simulink model "Two_Wheel_PI"  (R2021b)
settings: Solver=VariableStepAuto  StartTime=0.0  StopTime=10.0  RelTol=1e-3
model workspace (MAT data in the model file):
  Ki = 3
  Kp = 1
  ic = [0 0 0 0 0 0]
  param = [9.81 0.05 0.2 0.2 0.1 0.01 0.01 1 1 1 1 1 1]
undefined symbols (not defined in the file or in its folder): B_s
settings Model: Creator=Lorenzo  LastModifiedBy=Lorenzo

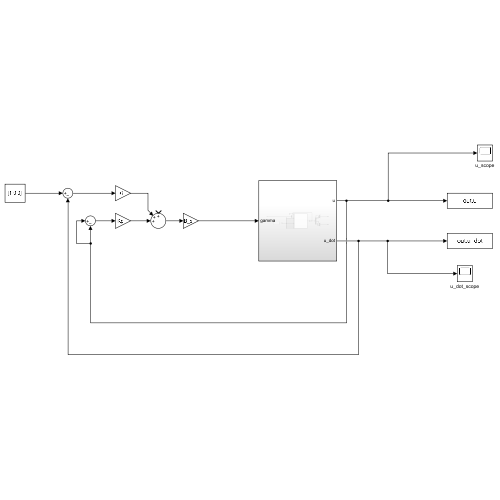
[thumbnail: Simulink's stored preview of the top-level diagram]
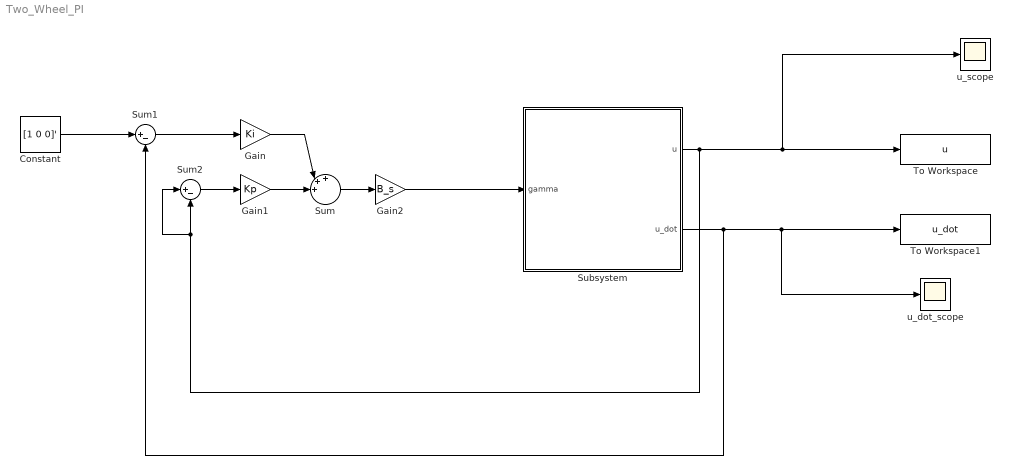
== system Two_Wheel_PI ==
  Constant : Constant  Value=[1 0 0]'
  Gain : Gain  Gain=Ki
  Gain1 : Gain  Gain=Kp
  Gain2 : Gain  Gain=B_s
  Subsystem : Subsystem
  Sum : Sum  Inputs=+++||
  Sum1 : Sum  Inputs=|+-
  Sum2 : Sum  Inputs=|+-
  To Workspace : ToWorkspace  VariableName=u  SaveFormat=Timeseries  SampleTime=-1
  To Workspace1 : ToWorkspace  VariableName=u_dot  SaveFormat=Timeseries  SampleTime=-1
  u_dot_scope : Scope
  u_scope : Scope
  wires:
  Subsystem/2(u_dot) -> u_dot_scope/1, To Workspace1/1, Sum1/2
  Subsystem/1(u) -> To Workspace/1, u_scope/1, Sum2/1, Sum2/2
  Gain2/1 -> Subsystem/1(gamma)
  Sum/1 -> Gain2/1
  Gain1/1 -> Sum/3
  Gain/1 -> Sum/2
  Sum1/1 -> Gain/1
  Sum2/1 -> Gain1/1
  Constant/1 -> Sum1/1

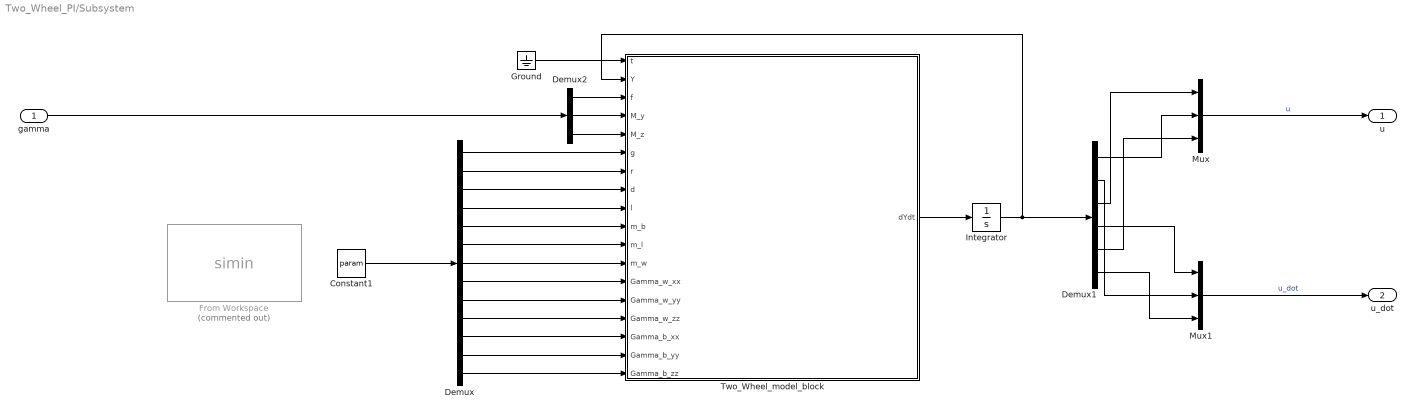
== system Two_Wheel_PI/Subsystem ==
  gamma : Inport
  Constant1 : Constant  Value=param
  Demux : Demux  Outputs=13
  Demux1 : Demux  Outputs=6
  Demux2 : Demux  Outputs=3
  From Workspace : FromWorkspace  Commented=on  VariableName=simin
  Ground : Ground
  Integrator : Integrator  InitialCondition=ic
  Mux : Mux  Inputs=3
  Mux1 : Mux  Inputs=3
  Two_Wheel_model_block : MATLAB Function  TreatAsAtomicUnit=on
  u : Outport
  u_dot : Outport  Port=2
  wires:
  Demux/9 -> Two_Wheel_model_block/14(Gamma_w_yy)
  Demux/13 -> Two_Wheel_model_block/18(Gamma_b_zz)
  Mux1/1 -> u_dot/1  "u_dot"
  Demux/12 -> Two_Wheel_model_block/17(Gamma_b_yy)
  Demux1/6 -> Mux1/3
  Demux/3 -> Two_Wheel_model_block/8(d)
  Demux1/5 -> Mux/3
  Demux2/2 -> Two_Wheel_model_block/4(M_y)
  gamma/1 -> Demux2/1
  Demux/2 -> Two_Wheel_model_block/7(r)
  Demux/8 -> Two_Wheel_model_block/13(Gamma_w_xx)
  Demux/10 -> Two_Wheel_model_block/15(Gamma_w_zz)
  Demux/5 -> Two_Wheel_model_block/10(m_b)
  Demux/4 -> Two_Wheel_model_block/9(l)
  Demux/6 -> Two_Wheel_model_block/11(m_l)
  Demux/11 -> Two_Wheel_model_block/16(Gamma_b_xx)
  Demux2/1 -> Two_Wheel_model_block/3(f)
  Demux/1 -> Two_Wheel_model_block/6(g)
  Demux/7 -> Two_Wheel_model_block/12(m_w)
  Demux2/3 -> Two_Wheel_model_block/5(M_z)
  Mux/1 -> u/1  "u"
  Constant1/1 -> Demux/1
  Ground/1 -> Two_Wheel_model_block/1(t)
  Integrator/1 -> Two_Wheel_model_block/2(Y), Demux1/1
  Two_Wheel_model_block/1(dYdt) -> Integrator/1
  Demux1/3 -> Mux/1
  Demux1/1 -> Mux/2
  Demux1/4 -> Mux1/1
  Demux1/2 -> Mux1/2

== matlab function Two_Wheel_PI/Subsystem/Two_Wheel_model_block ==
  data: t input; dYdt output; Y input; f input; M_y input; M_z input; g input; r input; d input; l input; m_b input; m_l input; m_w input; Gamma_w_xx input; Gamma_w_yy input; Gamma_w_zz input; Gamma_b_xx input; Gamma_b_yy input; Gamma_b_zz input
function dYdt = Two_Wheel_model_block(t,Y,f,M_y,M_z,g,r,d,l,m_b,m_l,m_w,Gamma_w_xx,Gamma_w_yy,Gamma_w_zz,Gamma_b_xx,Gamma_b_yy,Gamma_b_zz)
%#codegen

%    This function was generated by the Symbolic Math Toolbox version 9.0.
%    14-Sep-2022 15:36:12

t2 = Y(1);
t3 = d.^2;
t4 = l.^2;
t5 = m_w.^2;
t6 = r.^2;
t7 = Gamma_b_yy.*Gamma_w_yy;
t8 = sin(t2);
t9 = Gamma_w_yy.*m_w.*t4;
t10 = Gamma_b_yy.*m_w.*t6.*3.0;
t11 = t4.*t5.*t6.*2.0;
t12 = t7+t9+t10+t11;
t13 = 1.0./t12;
dYdt = [Y(2);t13.*(Gamma_w_yy.*M_y+M_y.*m_w.*t6.*3.0-f.*l.*m_w.*t6+Gamma_w_yy.*g.*l.*t8+g.*l.*m_w.*t6.*t8.*3.0);Y(4);t6.*t13.*(Gamma_b_yy.*f-M_y.*l.*m_w+f.*m_w.*t4-g.*m_w.*t4.*t8);Y(6);(M_z.*t6.*2.0)./(Gamma_b_zz.*t6.*2.0+Gamma_w_yy.*t3+Gamma_w_zz.*t6.*4.0+m_w.*t3.*t6)];
